simulink model "bomba"  (R2013a)
settings: Solver=ode45  StartTime=0.0  StopTime=1660  RelTol=1e-3
values from neighbouring files (symbols this model uses):
  C = 200    [bomba_consts.m]
  h_bar = 12    [bomba_consts.m]
  q_bar = 34.71    [bomba_consts.m]
  R = 1.0775    [bomba_consts.m]
settings Model: Creator=angel.garcia  LastModifiedBy=angel.garcia

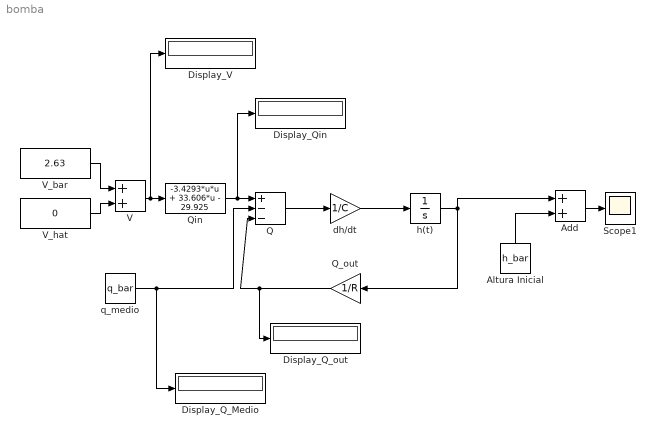
== system bomba ==
  Add : Sum
  Altura Inicial : Constant  Value=h_bar
  Display_Q_Medio : Display
  Display_Q_out : Display
  Display_Qin : Display
  Display_V : Display
  Q : Sum  Inputs=+--
  Q_out : Gain  Gain=1/R
  Qin : Fcn  Expr=-3.4293*u*u + 33.606*u - 29.925
  Scope1 : Scope
      settings: TimeRange=1660
  V : Sum
  V_bar : Constant  Value=2.63
  V_hat : Constant  Value=0
  dh/dt : Gain  Gain=1/C
  h(t) : Integrator
  q_medio : Constant  Value=q_bar
  wires:
  Q/1 -> dh/dt/1
  dh/dt/1 -> h(t)/1
  h(t)/1 -> Q_out/1, Add/1
  Q_out/1 -> Display_Q_out/1, Q/3
  Add/1 -> Scope1/1
  Altura Inicial/1 -> Add/2
  Qin/1 -> Display_Qin/1, Q/1
  q_medio/1 -> Display_Q_Medio/1, Q/2
  V/1 -> Display_V/1, Qin/1
  V_bar/1 -> V/1
  V_hat/1 -> V/2
